simulink model "Reconstruction_Circuit"  (R2020b)
settings: Solver=VariableStepAuto  StartTime=0.0  StopTime=43848  MaxStep=5/60  RelTol=1e-4
undefined symbols (not defined in the file): K, tau1, tau2
settings Model: Creator=andre  LastModifiedBy=andre

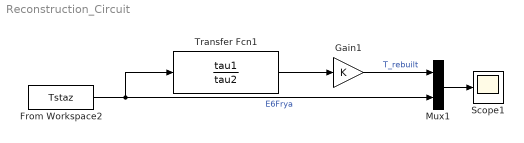
== system Reconstruction_Circuit ==
  From Workspace2 : FromWorkspace  VariableName=Tstaz  Interpolate=off  ZeroCross=off  OutputAfterFinalValue=Holding final value
  Gain1 : Gain  Gain=K
  Mux1 : Mux  Inputs=2
  Scope1 : Scope
  Transfer Fcn1 : TransferFcn  Numerator=tau1  Denominator=tau2
  wires:
  From Workspace2/1 -> Mux1/2, Transfer Fcn1/1  "E6Frya"
  Transfer Fcn1/1 -> Gain1/1
  Mux1/1 -> Scope1/1
  Gain1/1 -> Mux1/1  "T_rebuilt"
